simulink model "vehicle_animation_sim"  (Simulink 9.1)
settings: Solver=ode45  StartTime=0.0  StopTime=5  RelTol=1e-3
undefined symbols (not defined in the file): animation_update_interval, datetime, enable_CG_trace, enable_rearAxle_trace, plotAxisLimitMode, plotAxisLimits, save_anim_frames, vehicle_length, vehicle_width, X_ic, Y_ic, yaw_ic
settings Model: Creator=comperem  LastModifiedBy=fredd
settings DataIOCC: LimitDataPoints=on
settings OptimizationCC: BlockReduction=off  BooleanDataType=off
settings DebuggingCC: SaveWithParameterizedLinksMsg=none  SignalResolutionControl=TryResolveAllWithWarning  AllowSymbolicDim=off
settings HardwareCC: TargetUnknown=on
settings GRTTargetCC: GeneratePreprocessorConditionals=Disable all  CombineOutputUpdateFcns=on  GRTInterface=off
settings ConfigComp: CovSFcnEnable=off

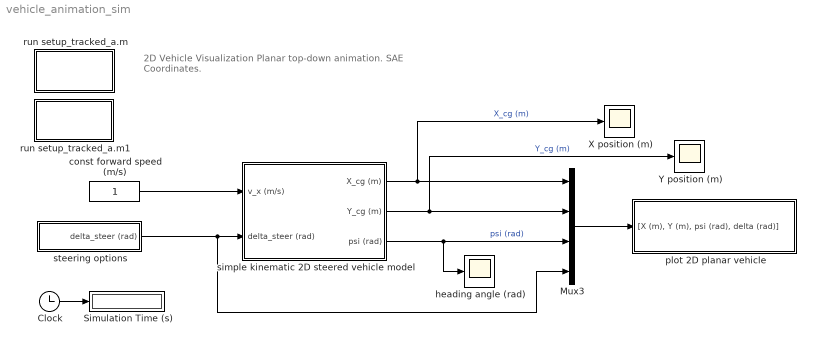
== system vehicle_animation_sim ==
  note: 2D Vehicle Visualization
      | Planar top-down animation.
      | SAE Coordinates.
  Clock : Clock
  Mux3 : Mux
  Simulation Time (s) : Display
  X position (m) : Scope
  Y position (m) : Scope
  const forward speed (m/s) : Constant
  heading angle (rad) : Scope
  plot 2D planar vehicle : Subsystem  mask(6DoF Animation){axisMode=plotAxisLimitMode, ax=plotAxisLimits, Ts=animation_update_interval, enable_CG_trace=enable_CG_trace, enable_rearAxle_trace=enable_rearAxle_trace, save_anim_frames=save_anim_frames, anim_frame_name_str=char(datetime('now','Format','yyyy-MM-dd_HH_mm_ss')), L=vehicle_length, W=vehicle_width}
      mask prompts: axisMode "Axis Mode (0->auto, 1->fixed, BOTH use Axes Limits below)"; ax "Axes limits [xmin xmax ymin ymax] (m):"; Ts "Time interval between updates (s):"; enable_CG_trace "Enable vehicle CG trace? (0/1)"; enable_rearAxle_trace "Enable rear axle trace? (0/1)"; save_anim_frames "Save animaton frames? (0/1)"; anim_frame_name_str "Animation sequence name (if save frames==1)"; L "Vehicle length (m)"; W "Vehicle width (m)"
      mask help:
      | Create a 2D animated view of a steering vehicle model with tires.
      |
      | Marc Compere
      | CompereM@saic.com
      | created : 22 August 2002
      | modified: 28 Dec 2015
      mask init:
      | Config.axisMode=axisMode;
      | Config.ax=ax;
      | Config.Ts=Ts;
      | Config.enable_CG_trace=enable_CG_trace;
      | Config.enable_rearAxle_trace=enable_rearAxle_trace;
      | Config.save_anim_frames=save_anim_frames;
      | Config.anim_frame_name_str=anim_frame_name_str;
      | Config.L=L;
      | Config.W=W;
      mask Help:
      | <p>This block generates a 3 dimensional display of a simulation trajectory, with the craft orientation displayed during flight</p>
      | 
      | <p>There are two inputs to this block, Position and Euler.  These inputs contain more than one signal as described below.</p>
      | 
      | <p><H4>Block Vector Input - Position</H4>
      | <ul>
      | <li>X Position</li>
      | <li>Y Position</li>
      | <li>Z Position</li>
      | </ul>
      | </p>
      | 
      | <p><H4>Block Vector Input - Euler</H4>
      |     <ul>
      |     <li>Roll Attitude</li>
      |     <li>Pitch Attitude</li>
      |     <li>Yaw Attitude</li>
      |    </ul>
      |    </p>
  run setup_tracked_a.m : Subsystem
      settings: OpenFcn=setup
      mask Display: fprintf('run setup.m')
  run setup_tracked_a.m1 : Subsystem
      settings: OpenFcn=edit setup
      mask Display: fprintf('edit setup.m')
  simple kinematic 2D steered vehicle model : Subsystem
  steering options : Subsystem
  wires:
  simple kinematic 2D steered vehicle model/1(X_cg (m)) -> Mux3/1, X position (m)/1  "X_cg (m)"
  simple kinematic 2D steered vehicle model/2(Y_cg (m)) -> Y position (m)/1, Mux3/2  "Y_cg (m)"
  simple kinematic 2D steered vehicle model/3(psi (rad)) -> heading angle (rad)/1, Mux3/3  "psi (rad)"
  Clock/1 -> Simulation Time (s)/1
  const forward speed (m/s)/1 -> simple kinematic 2D steered vehicle model/1(v_x (m/s))
  Mux3/1 -> plot 2D planar vehicle/1("[X (m), Y (m), psi (rad), delta (rad)]")
  steering options/1(delta_steer (rad)) -> Mux3/4, simple kinematic 2D steered vehicle model/2(delta_steer (rad))

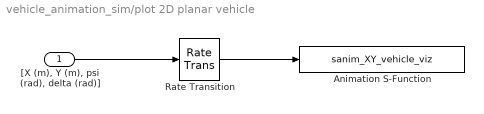
== system vehicle_animation_sim/plot 2D planar vehicle ==
  "[X (m), Y (m), psi (rad), delta (rad)]" : Inport
  Animation S-Function : S-Function  FunctionName=sanim_XY_vehicle_viz  Parameters=Config  SFunctionDeploymentMode=off  EnableBusSupport=off
  Rate Transition : RateTransition  Integrity=off
  wires:
  "[X (m), Y (m), psi (rad), delta (rad)]"/1 -> Rate Transition/1
  Rate Transition/1 -> Animation S-Function/1

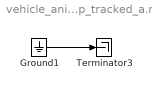
== system vehicle_animation_sim/run setup_tracked_a.m ==
  Ground1 : Ground
  Terminator3 : Terminator
  wires:
  Ground1/1 -> Terminator3/1

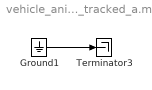
== system vehicle_animation_sim/run setup_tracked_a.m1 ==
  Ground1 : Ground
  Terminator3 : Terminator
  wires:
  Ground1/1 -> Terminator3/1

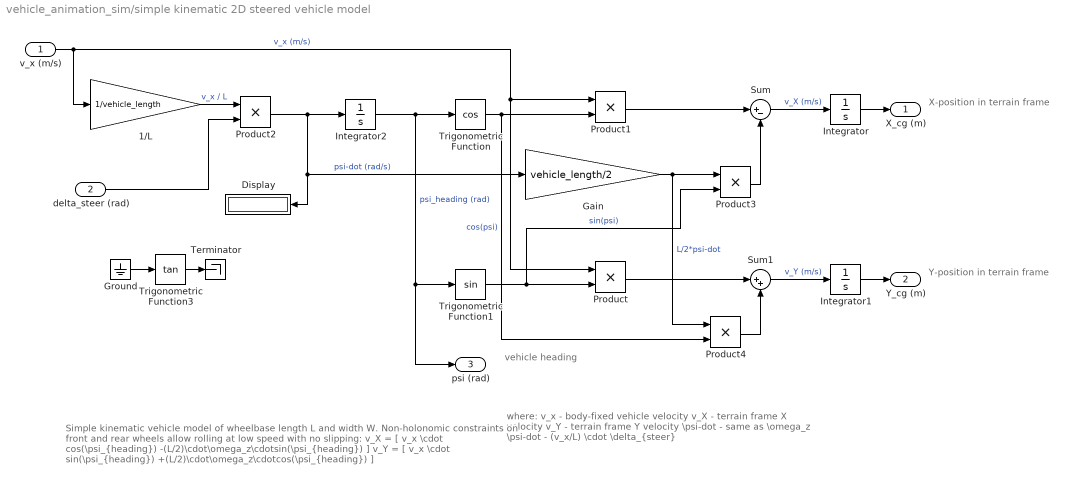
== system vehicle_animation_sim/simple kinematic 2D steered vehicle model ==
  note: where:
      |    v_x - body-fixed vehicle velocity
      |    v_X - terrain frame X velocity
      |    v_Y - terrain frame Y velocity
      |    \psi-dot - same as \omega_z
      |    \psi-dot - (v_x/L) \cdot \delta_{steer}
  note: X-position in
      | terrain frame
  note: Simple kinematic vehicle model of wheelbase
      | length L and width W.
      | Non-holonomic constraints on front and rear wheels
      | allow rolling at low speed with no slipping:
      |
      |    v_X = [ v_x \cdot cos(\psi_{heading}) -(L/2)\cdot\omega_z\cdotsin(\psi_{heading}) ]
      |    v_Y = [ v_x \cdot sin(\psi_{heading}) +(L/2)\cdot\omega_z\cdotcos(\psi_{heading}) ]
  note: vehicle
      | heading
  note: Y-position in
      | terrain frame
  v_x (m/s) : Inport
  delta_steer (rad) : Inport  Port=2
  1/L : Gain  Gain=1/vehicle_length
  Display : Display
  Gain : Gain  Gain=vehicle_length/2
  Ground : Ground
  Integrator : Integrator  InitialCondition=X_ic
  Integrator1 : Integrator  InitialCondition=Y_ic
  Integrator2 : Integrator  InitialCondition=yaw_ic
  Product{,1..4} (5 alike) : Product  RndMeth=Zero
  Sum : Sum  Inputs=|+-
  Sum1 : Sum  Inputs=|++
  Terminator : Terminator
  Trigonometric Function : Trigonometry  Operator=cos
  Trigonometric Function1 : Trigonometry
  Trigonometric Function3 : Trigonometry  Operator=tan
  X_cg (m) : Outport
  Y_cg (m) : Outport  Port=2
  psi (rad) : Outport  Port=3
  wires:
  Product/1 -> Sum1/1
  Product1/1 -> Sum/1
  Trigonometric Function/1 -> Product4/2, Product1/2  "cos(psi)"
  Trigonometric Function1/1 -> Product/2, Product3/2  "sin(psi)"
  Integrator2/1 -> Trigonometric Function/1, Trigonometric Function1/1, psi (rad)/1  "psi_heading (rad)"
  Integrator/1 -> X_cg (m)/1
  Integrator1/1 -> Y_cg (m)/1
  v_x (m/s)/1 -> Product/1, Product1/1, 1/L/1  "v_x (m/s)"
  Product2/1 -> Gain/1, Display/1, Integrator2/1  "psi-dot (rad/s)"
  1/L/1 -> Product2/1  "v_x / L"
  Sum/1 -> Integrator/1  "v_X (m/s)"
  Sum1/1 -> Integrator1/1  "v_Y (m/s)"
  Gain/1 -> Product4/1, Product3/1  "L/2*psi-dot"
  Product3/1 -> Sum/2
  Product4/1 -> Sum1/2
  delta_steer (rad)/1 -> Product2/2
  Ground/1 -> Trigonometric Function3/1
  Trigonometric Function3/1 -> Terminator/1

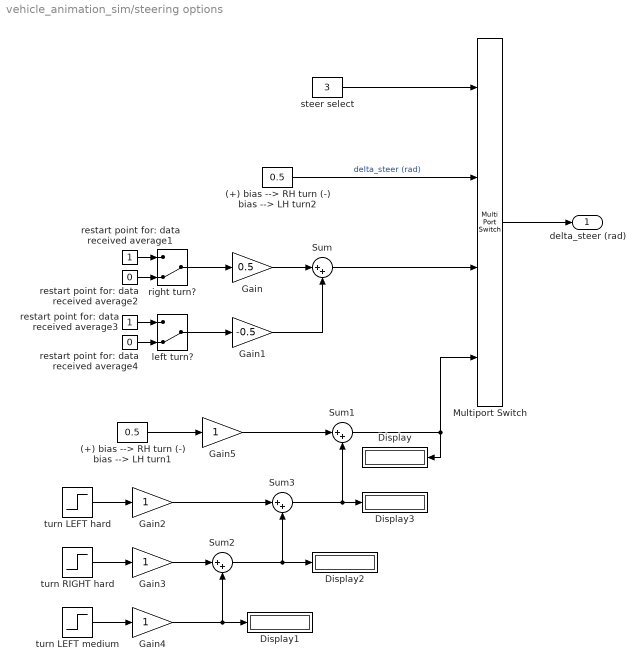
== system vehicle_animation_sim/steering options ==
  (+) bias --> RH turn (-) bias --> LH turn1 : Constant  Value=0.5
  (+) bias --> RH turn (-) bias --> LH turn2 : Constant  Value=0.5
  Display{,1..3} (4 alike) : Display
  Gain : Gain  Gain=0.5
  Gain1 : Gain  Gain=-0.5
  Gain{2..5} (4 alike) : Gain
  Multiport Switch : MultiPortSwitch
  Sum{,1..3} (4 alike) : Sum  Inputs=|++
  left turn? : ManualSwitch  CurrentSetting=0
  restart point for: data received average1 : Constant
  restart point for: data received average2 : Constant  Value=0
  restart point for: data received average3 : Constant
  restart point for: data received average4 : Constant  Value=0
  right turn? : ManualSwitch  CurrentSetting=0
  steer select : Constant  Value=3
  turn LEFT hard : Step  Time=10  After=-1  SampleTime=0
  turn LEFT medium : Step  Time=30  After=-0.5  SampleTime=0
  turn RIGHT hard : Step  Time=20  After=+1  SampleTime=0
  delta_steer (rad) : Outport
  wires:
  (+) bias --> RH turn (-) bias --> LH turn2/1 -> Multiport Switch/2  "delta_steer (rad)"
  steer select/1 -> Multiport Switch/1
  Multiport Switch/1 -> delta_steer (rad)/1
  restart point for: data received average1/1 -> right turn?/1
  restart point for: data received average2/1 -> right turn?/2
  Sum/1 -> Multiport Switch/3
  right turn?/1 -> Gain/1
  restart point for: data received average3/1 -> left turn?/1
  restart point for: data received average4/1 -> left turn?/2
  left turn?/1 -> Gain1/1
  Gain/1 -> Sum/1
  Gain1/1 -> Sum/2
  Sum1/1 -> Multiport Switch/4, Display/1
  (+) bias --> RH turn (-) bias --> LH turn1/1 -> Gain5/1
  turn RIGHT hard/1 -> Gain3/1
  turn LEFT medium/1 -> Gain4/1
  turn LEFT hard/1 -> Gain2/1
  Sum2/1 -> Display2/1, Sum3/2
  Sum3/1 -> Display3/1, Sum1/2
  Gain2/1 -> Sum3/1
  Gain3/1 -> Sum2/1
  Gain4/1 -> Display1/1, Sum2/2
  Gain5/1 -> Sum1/1
